simulink model "Hybrid_vehicle"  (R2020a)
settings: Solver=VariableStepAuto  StartTime=0.0  StopTime=1800  MaxStep=0.05  RelTol=1e-8
values from neighbouring files (symbols this model uses):
  Bdy_facTireFric_C = 0.018    [Model_parameters.mat]
  Bdy_lenRadiusWheel_C = 0.32    [Model_parameters.mat]
  Bdy_mEquivalentJ_C = 60    [Model_parameters.mat]
  Bdy_mVeh_C = 1400    [Model_parameters.mat]
  Bdy_vsqr2frc_C = 0.429    [Model_parameters.mat]
  Drv_facSlopeWLTC_CUR = [0 500 1000 1500 2000 2500 3000 3500 4000 4500 5000 5500 ... (98 elements, 49x2)]    [Model_parameters.mat]
  Drv_kmh2gradtqDriver_C = 200    [Model_parameters.mat]
  Drv_kmh2tqDriver_C = 500    [Model_parameters.mat]
  Drv_kmhDesWLTC_CUR = [1 2 3 4 5 6 7 8 9 10 11 12 ... (3600 elements, 1800x2)]    [Model_parameters.mat]
  Edr_pwr_LossMap_AXIS = [-150000 -100000 -60000 -35000 -23000 -7000 -2000 -1000 -200 0 200 1000 ... (19 elements, 1x19)]    [Model_parameters.mat]
  Edr_pwrInverterLosses_MAP = [19500 13000 6600 3500 2990 1470 600 450 160 50 160 450 ... (76 elements, 19x4)]    [Model_parameters.mat]
  Edr_pwrMachineLosses_MAP = [330 270 210 150 120 90 60 30 10 0 20 40 ... (209 elements, 19x11)]    [Model_parameters.mat]
  Edr_rpm_InvLossMap_AXIS = [0 2000 5000 12000]    [Model_parameters.mat]
  Edr_rpm_MachLossMap_AXIS = [0 100 200 400 1000 2000 4000 6000 8000 10000 12000]    [Model_parameters.mat]
  Edr_rpm_MaxMinTq_AXIS = [0 100 200 400 1000 2000 4000 5000 6000 7000 8000 10000 ... (13 elements, 13x1)]    [Model_parameters.mat]
  Edr_tq_MachLossMap_AXIS = [-220 -180 -140 -100 -80 -60 -40 -20 -10 0 10 20 ... (19 elements, 1x19)]    [Model_parameters.mat]
  Edr_tqEffMax_CUR = [220 220 220 220 220 220 220 180 150 125 106 81 ... (13 elements, 13x1)]    [Model_parameters.mat]
  GbxFr_tqClutchMax_C = 500    [Model_parameters.mat]
  GbxRe_facGbxReRatio_C = 10    [Model_parameters.mat]
  Ice_derfacLoadDecrease_MAP = [-5 -200 -225 -250 -275 -300 -325 -350 -375 -400 -10 -400 ... (120 elements, 10x12)]    [Model_parameters.mat]
  Ice_derfacLoadIncrease_MAP = [500 30 30 30 30 30 0 0 0 0 500 50 ... (120 elements, 10x12)]    [Model_parameters.mat]
  Ice_facEtaCocMax_MAP = [1 1 0.98 0.955 0.93 1 1 0.986 0.965 0.94 1 1 ... (35 elements, 5x7)]    [Model_parameters.mat]
  Ice_facFuelEnRich_MAP = [1 1 1 1 1 1 1 1 1 1.02 1 1 ... (35 elements, 5x7)]    [Model_parameters.mat]
  Ice_Load2TqOptIgnLamOne_MAP = [0 35 70 105 140 0 38 76 114 152 0 40 ... (35 elements, 5x7)]    [Model_parameters.mat]
  Ice_relLoad_AXIS = [0 40 80 120 160]    [Model_parameters.mat]
  Ice_relLoad_LoadDyn_AXIS = [0 80 90 100 110 120 130 140 150 160]    [Model_parameters.mat]
  Ice_relLoad_Max_CUR = [50 130 137 143 148 153 159 160 160 157 130 90]    [Model_parameters.mat]
  Ice_rpm_AXIS = [0 1000 2000 3000 4000 5000 6000]    [Model_parameters.mat]
  Ice_rpm_LoadDyn_AXIS = [500 1000 1100 1200 1300 1400 1600 2400 3000 4000 5000 6000]    [Model_parameters.mat]
  Ice_tq_AXIS = [0 40 80 120 160]    [Model_parameters.mat]
  Ice_tqLossesIce_MAP = [15 13 11 11 11 15 13 11 11 11 16 14 ... (35 elements, 5x7)]    [Model_parameters.mat]
  Ice_TqOptIgnLamOne2Load_MAP = [0 45.7 91.4 137.14 182.85 0 42.1 84.2 126.3 168.4 0 40 ... (35 elements, 5x7)]    [Model_parameters.mat]
  Pnt_capBat_C = 54000    [Model_parameters.mat]
  Pnt_facSocInit_C = 0.6    [Model_parameters.mat]
  Pnt_resBatInner_C = 0.2    [Model_parameters.mat]
libraries: simulink x2
(part 1 of 2)
settings Model: SimulationMode=accelerator  Creator=Georg  LastModifiedBy=frank
settings DataIOCC: OutputSaveName=simout  ReturnWorkspaceOutputsName=simout
settings DebuggingCC: ArithmeticOperatorsInVariantConditions=warning
settings SFSimCC: CustomCodeUndefinedFunction=UseInterfaceOnly

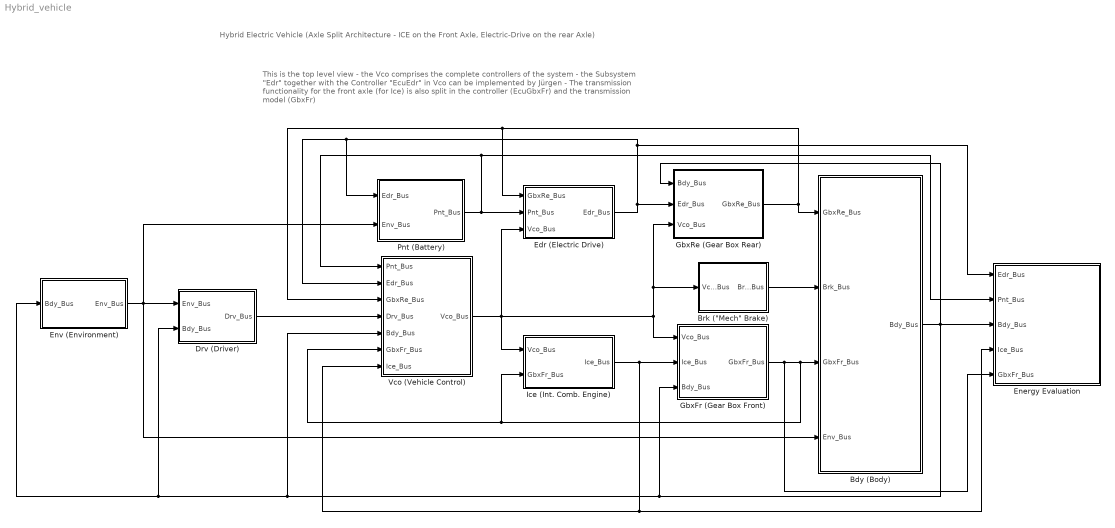
== system Hybrid_vehicle ==
  note: This is the top level view
      | - the Vco comprises the complete controllers of the system
      | - the Subsystem "Edr" together with the Controller "EcuEdr" in Vco can be implemented by Jürgen
      | - The transmission functionality for the front axle (for Ice) is also split in the controller (EcuGbxFr) and the transmission model (GbxFr)
  note: Hybrid Electric Vehicle (Axle Split Architecture - ICE on the Front Axle, Electric-Drive on the rear Axle)
  Bdy (Body) : Subsystem
      mask Display: image('Car_Top.png'); % Use "Edit Image" on toolstrip to change.
  "Brk (\"Mech\" Brake)" : Subsystem
      mask Display: image('Brakes.jpg'); % Use "Edit Image" on toolstrip to change.
  Drv (Driver) : Subsystem
      mask Display: image('Driver.jpg'); % Use "Edit Image" on toolstrip to change.
  Edr (Electric Drive) : Subsystem
      mask Display: image('e-motor.jpg'); % Use "Edit Image" on toolstrip to change.
  Energy Evaluation : Subsystem
      mask Display: image('Evaluation.png'); % Use "Edit Image" on toolstrip to change.
  Env (Environment) : Subsystem
      mask Display: image('Environment.jpg'); % Use "Edit Image" on toolstrip to change.
  GbxFr (Gear Box Front) : Subsystem
      mask Display: image('Gearbox.jpg'); % Use "Edit Image" on toolstrip to change.
  GbxRe (Gear Box Rear) : Subsystem
      mask Display: image('Gearbox.jpg'); % Use "Edit Image" on toolstrip to change.
  Ice (Int. Comb. Engine) : Subsystem
      mask Display: image('ICEngine.jpg'); % Use "Edit Image" on toolstrip to change.
  Pnt (Battery) : Subsystem
      mask Display: image('Battery.jpg'); % Use "Edit Image" on toolstrip to change.
  Vco (Vehicle Control) : Subsystem
      mask Display: image('VehicleControlUnit.jpg'); % Use "Edit Image" on toolstrip to change.
  wires:
  Drv (Driver)/1(Drv_Bus) -> Vco (Vehicle Control)/4(Drv_Bus)
  Env (Environment)/1(Env_Bus) -> Bdy (Body)/4(Env_Bus), Drv (Driver)/1(Env_Bus), Pnt (Battery)/2(Env_Bus)
  Vco (Vehicle Control)/1(Vco_Bus) -> Edr (Electric Drive)/3(Vco_Bus), Ice (Int. Comb. Engine)/1(Vco_Bus), GbxFr (Gear Box Front)/1(Vco_Bus), GbxRe (Gear Box Rear)/3(Vco_Bus), "Brk (\"Mech\" Brake)"/1(Vco_Bus)
  Pnt (Battery)/1(Pnt_Bus) -> Edr (Electric Drive)/2(Pnt_Bus), Vco (Vehicle Control)/1(Pnt_Bus), Energy Evaluation/2(Pnt_Bus)
  Edr (Electric Drive)/1(Edr_Bus) -> GbxRe (Gear Box Rear)/2(Edr_Bus), Pnt (Battery)/1(Edr_Bus), Vco (Vehicle Control)/2(Edr_Bus), Energy Evaluation/1(Edr_Bus)
  Ice (Int. Comb. Engine)/1(Ice_Bus) -> Energy Evaluation/4(Ice_Bus), Vco (Vehicle Control)/7(Ice_Bus), GbxFr (Gear Box Front)/2(Ice_Bus)
  GbxRe (Gear Box Rear)/1(GbxRe_Bus) -> Bdy (Body)/1(GbxRe_Bus), Edr (Electric Drive)/1(GbxRe_Bus), Vco (Vehicle Control)/3(GbxRe_Bus)
  GbxFr (Gear Box Front)/1(GbxFr_Bus) -> Energy Evaluation/5(GbxFr_Bus), Vco (Vehicle Control)/6(GbxFr_Bus), Ice (Int. Comb. Engine)/2(GbxFr_Bus), Bdy (Body)/3(GbxFr_Bus)
  "Brk (\"Mech\" Brake)"/1(Brk_Bus) -> Bdy (Body)/2(Brk_Bus)
  Bdy (Body)/1(Bdy_Bus) -> GbxRe (Gear Box Rear)/1(Bdy_Bus), Energy Evaluation/3(Bdy_Bus), GbxFr (Gear Box Front)/3(Bdy_Bus), Vco (Vehicle Control)/5(Bdy_Bus), Env (Environment)/1(Bdy_Bus), Drv (Driver)/2(Bdy_Bus)

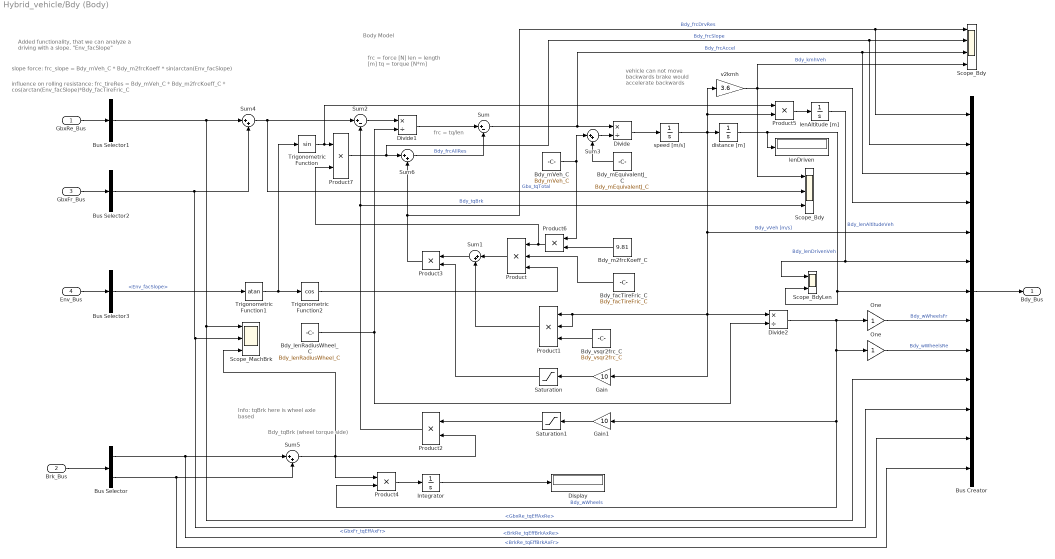
== system Hybrid_vehicle/Bdy (Body) ==
  note: influence on rolling resistance: frc_tireRes = Bdy_mVeh_C * Bdy_m2frcKoeff_C * cos(arctan(Env_facSlope)*Bdy_facTireFric_C
  note: slope force: frc_slope = Bdy_mVeh_C * Bdy_m2frcKoeff * sin(arctan(Env_facSlope)
  note: Added functionality, that we can analyze a
      | driving with a slope.  "Env_facSlope"
  note: Body Model
  note: Info:
      | tqBrk here is wheel axle based
  note: Bdy_tqBrk
      | (wheel torque side)
  note: frc = force [N]
      | len = length [m]
      | tq = torque [N*m]
  note: vehicle can not
      | move backwards
      | brake would accelerate
      | backwards
  note: frc = tq/len
  GbxRe_Bus : Inport
  Brk_Bus : Inport  Port=2
  GbxFr_Bus : Inport  Port=3
  Env_Bus : Inport  Port=4
  Bdy_facTireFric_C : Constant  Value=Bdy_facTireFric_C
  Bdy_lenRadiusWheel_C : Constant  Value=Bdy_lenRadiusWheel_C
  Bdy_m2frcKoeff_C : Constant  Value=9.81
  Bdy_mEquivalentJ_C : Constant  Value=Bdy_mEquivalentJ_C
  Bdy_mVeh_C : Constant  Value=Bdy_mVeh_C
  Bdy_vsqr2frc_C : Constant  Value=Bdy_vsqr2frc_C
  Bus Creator : BusCreator  Inputs=13
  Bus Selector : BusSelector  OutputSignals=BrkRe_tqEffBrkAxRe,BrkRe_tqEffBrkAxFr
  Bus Selector1 : BusSelector  OutputSignals=GbxRe_tqEffAxRe
  Bus Selector2 : BusSelector  OutputSignals=GbxFr_tqEffAxFr
  Bus Selector3 : BusSelector  OutputSignals=Env_facSlope
  Display : Display
  Divide : Product  Inputs=*/
  Divide1 : Product  Inputs=*/
  Divide2 : Product  Inputs=*/
  Gain : Gain  Gain=10
  Gain1 : Gain  Gain=10
  Integrator : Integrator
  One : Gain
  "One " : Gain
  Product : Product  Inputs=3  RndMeth=Zero
  Product1 : Product  Inputs=3  RndMeth=Zero
  Product2 : Product  RndMeth=Zero
  Product3 : Product  RndMeth=Zero
  Product4 : Product
  Product5 : Product
  Product6 : Product  RndMeth=Zero
  Product7 : Product
  Saturation : Saturate  UpperLimit=1  LowerLimit=-1
  Saturation1 : Saturate  UpperLimit=1  LowerLimit=-1
  Scope_Bdy : Scope  NumInputPorts=3
  "Scope_Bdy " : Scope  NumInputPorts=4
  "Scope_BdyLen  " : Scope  NumInputPorts=2
  Scope_MachBrk : Scope  NumInputPorts=3
  Sum : Sum  Inputs=|+-
  Sum{1,3..6} (5 alike) : Sum  Inputs=|++
  Sum2 : Sum  Inputs=|+-
  Trigonometric Function : Trigonometry
  Trigonometric Function1 : Trigonometry  Operator=atan
  Trigonometric Function2 : Trigonometry  Operator=cos
  distance [m] : Integrator
  lenAltitude [m] : Integrator
  lenDriven : Display
  speed [m/s] : Integrator  LimitOutput=on  LowerSaturationLimit=0
  v2kmh : Gain  Gain=3.6
  Bdy_Bus : Outport  VectorParamsAs1DForOutWhenUnconnected=off
  wires:
  Bus Creator/1 -> Bdy_Bus/1
  v2kmh/1 -> Bus Creator/4, Scope_Bdy/1, "Scope_Bdy "/4  "Bdy_kmhVeh"
  distance [m]/1 -> "Scope_BdyLen  "/2, Bus Creator/7, lenDriven/1  "Bdy_lenDrivenVeh"
  GbxFr_Bus/1 -> Bus Selector2/1
  GbxRe_Bus/1 -> Bus Selector1/1
  Brk_Bus/1 -> Bus Selector/1
  Bus Selector/1 -> Bus Creator/12, Sum5/1  "<BrkRe_tqEffBrkAxRe>"
  Bus Selector/2 -> Bus Creator/13, Sum5/2  "<BrkRe_tqEffBrkAxFr>"
  Saturation/1 -> Product3/2
  Bdy_m2frcKoeff_C/1 -> Product6/2
  Bdy_vsqr2frc_C/1 -> Product1/3
  Divide1/1 -> Sum/1
  Sum3/1 -> Divide/2
  Bdy_facTireFric_C/1 -> Product/2
  Gain/1 -> Saturation/1
  Sum/1 -> Divide/1, Bus Creator/3, "Scope_Bdy "/3  "Bdy_frcAccel"
  Gain1/1 -> Saturation1/1
  Sum5/1 -> Product2/2, Product4/1, Scope_MachBrk/3
  Sum2/1 -> Divide1/1
  Product2/1 -> Sum2/2, Scope_Bdy/3  "Bdy_tqBrk"
  Sum4/1 -> Sum2/1, Scope_Bdy/2  "Gbx_tqTotal"
  Bdy_lenRadiusWheel_C/1 -> Divide2/2, Divide1/2
  Sum1/1 -> Product3/1
  Bdy_mVeh_C/1 -> Product6/1, Sum3/1
  Product1/1 -> Sum1/2
  Divide/1 -> speed [m/s]/1
  speed [m/s]/1 -> Product5/2, v2kmh/1, distance [m]/1, Product1/1, Product1/2, Gain/1, Divide2/1, Bus Creator/5  "Bdy_vVeh [m/s]"
  Product3/1 -> Sum6/2, Bus Creator/1, "Scope_Bdy "/1  "Bdy_frcDrvRes"
  Divide2/1 -> One/1, Product4/2, Gain1/1, "One "/1  "Bdy_wWheels"
  Saturation1/1 -> Product2/1
  Bdy_mEquivalentJ_C/1 -> Sum3/2
  Bus Selector1/1 -> Sum4/1, Bus Creator/10, Scope_MachBrk/1  "<GbxRe_tqEffAxRe>"
  Bus Selector2/1 -> Sum4/2, Bus Creator/11, Scope_MachBrk/2  "<GbxFr_tqEffAxFr>"
  One/1 -> Bus Creator/9  "Bdy_wWheelsRe"
  "One "/1 -> Bus Creator/8  "Bdy_wWheelsFr"
  Product4/1 -> Integrator/1
  Integrator/1 -> Display/1
  Env_Bus/1 -> Bus Selector3/1
  Bus Selector3/1 -> Trigonometric Function1/1  "<Env_facSlope>"
  Trigonometric Function1/1 -> Trigonometric Function2/1, Trigonometric Function/1
  Trigonometric Function2/1 -> Product/3
  Sum6/1 -> Sum/2  "Bdy_frcAllRes"
  Product6/1 -> Product7/2, Product/1
  Product/1 -> Sum1/1
  Product7/1 -> Bus Creator/2, "Scope_Bdy "/2, Sum6/1  "Bdy_frcSlope"
  Trigonometric Function/1 -> Product5/1, Product7/1
  Product5/1 -> lenAltitude [m]/1
  lenAltitude [m]/1 -> "Scope_BdyLen  "/1, Bus Creator/6  "Bdy_lenAltitudeVeh"

== system Hybrid_vehicle/Brk ("Mech" Brake) ==
  note: Mechanical Brake Model
      | (both Axles)
  note: Info:
      | tq here is wheel axle based
  note: - very simple here, but a dynamik brake is not needed here
  Vco_Bus : Inport
  Bus Creator : BusCreator  Inputs=2
  Bus Selector : BusSelector  OutputSignals=EcuBrk_Bus
  Bus Selector1 : BusSelector  OutputSignals=EcuBrk_tqEffBrkAxReDes,EcuBrk_tqEffBrkAxFrDes
  Gain : Gain
  Gain1 : Gain
  Brk_Bus : Outport  VectorParamsAs1DForOutWhenUnconnected=off
  wires:
  Vco_Bus/1 -> Bus Selector/1
  Bus Selector/1 -> Bus Selector1/1  "<EcuBrk_Bus>"
  Bus Selector1/1 -> Gain/1  "<EcuBrk_tqEffBrkAxReDes>"
  Bus Selector1/2 -> Gain1/1  "<EcuBrk_tqEffBrkAxFrDes>"
  Bus Creator/1 -> Brk_Bus/1
  Gain/1 -> Bus Creator/1  "BrkRe_tqEffBrkAxRe"
  Gain1/1 -> Bus Creator/2  "BrkRe_tqEffBrkAxFr"

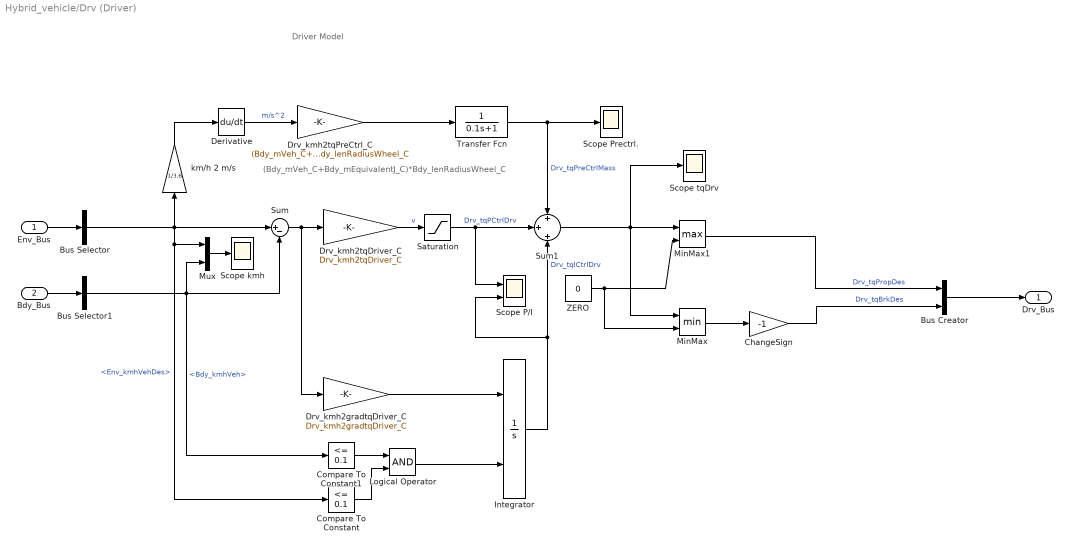
== system Hybrid_vehicle/Drv (Driver) ==
  note: (Bdy_mVeh_C+Bdy_mEquivalentJ_C)*Bdy_lenRadiusWheel_C
  note: Driver Model
  Env_Bus : Inport
  Bdy_Bus : Inport  Port=2
  Bus Creator : BusCreator  Inputs=2
  Bus Selector : BusSelector  OutputSignals=Env_kmhVehDes
  Bus Selector1 : BusSelector  OutputSignals=Bdy_kmhVeh
  ChangeSign : Gain  Gain=-1
  Compare To Constant : simulink/Logic and Bit Operations/Compare To Constant  relop=<=  const=0.1  OutDataTypeStr=boolean
  Compare To Constant1 : simulink/Logic and Bit Operations/Compare To Constant  relop=<=  const=0.1  OutDataTypeStr=boolean
  Derivative : Derivative  CoefficientInTFapproximation=0.1
  Drv_kmh2gradtqDriver_C : Gain  Gain=Drv_kmh2gradtqDriver_C
  Drv_kmh2tqDriver_C : Gain  Gain=Drv_kmh2tqDriver_C
  Drv_kmh2tqPreCtrl_C : Gain  Gain=(Bdy_mVeh_C+Bdy_mEquivalentJ_C)*Bdy_lenRadiusWheel_C
  Integrator : Integrator  ExternalReset=level  InitialCondition=-10  LimitOutput=on  UpperSaturationLimit=1000  LowerSaturationLimit=-1000
  Logical Operator : Logic  AllPortsSameDT=off  OutDataTypeStr=boolean
  MinMax : MinMax  Inputs=2
  MinMax1 : MinMax  Function=max  Inputs=2
  Mux : Mux  Inputs=2
  Saturation : Saturate  UpperLimit=1000  LowerLimit=-1000
  Scope P/I : Scope  NumInputPorts=2
  Scope Prectrl. : Scope
  Scope kmh : Scope
  Scope tqDrv : Scope
  Sum : Sum  Inputs=|+-
  Sum1 : Sum  Inputs=+|+|+
  Transfer Fcn : TransferFcn  Denominator=[0.1 1]
  ZERO : Constant  Value=0
  km/h 2 m/s : Gain  Gain=1/3.6
  Drv_Bus : Outport  VectorParamsAs1DForOutWhenUnconnected=off
  wires:
  Bus Creator/1 -> Drv_Bus/1
  MinMax1/1 -> Bus Creator/1  "Drv_tqPropDes"
  ChangeSign/1 -> Bus Creator/2  "Drv_tqBrkDes"
  Env_Bus/1 -> Bus Selector/1
  Bus Selector/1 -> Sum/1, km/h 2 m/s/1, Compare To Constant/1, Mux/1  "<Env_kmhVehDes>"
  Bdy_Bus/1 -> Bus Selector1/1
  Bus Selector1/1 -> Mux/2, Compare To Constant1/1, Sum/2  "<Bdy_kmhVeh>"
  Drv_kmh2gradtqDriver_C/1 -> Integrator/1
  ZERO/1 -> MinMax1/2, MinMax/2
  Drv_kmh2tqDriver_C/1 -> Saturation/1  "v"
  MinMax/1 -> ChangeSign/1
  Integrator/1 -> Sum1/3, Scope P/I/2  "Drv_tqICtrlDrv"
  Sum/1 -> Drv_kmh2tqDriver_C/1, Drv_kmh2gradtqDriver_C/1
  Sum1/1 -> Scope tqDrv/1, MinMax/1, MinMax1/1
  Mux/1 -> Scope kmh/1
  Derivative/1 -> Drv_kmh2tqPreCtrl_C/1  "m/s^2"
  Drv_kmh2tqPreCtrl_C/1 -> Transfer Fcn/1
  km/h 2 m/s/1 -> Derivative/1
  Transfer Fcn/1 -> Sum1/1, Scope Prectrl./1  "Drv_tqPreCtrlMass"
  Compare To Constant/1 -> Logical Operator/2
  Compare To Constant1/1 -> Logical Operator/1
  Logical Operator/1 -> Integrator/2
  Saturation/1 -> Sum1/2, Scope P/I/1  "Drv_tqPCtrlDrv"

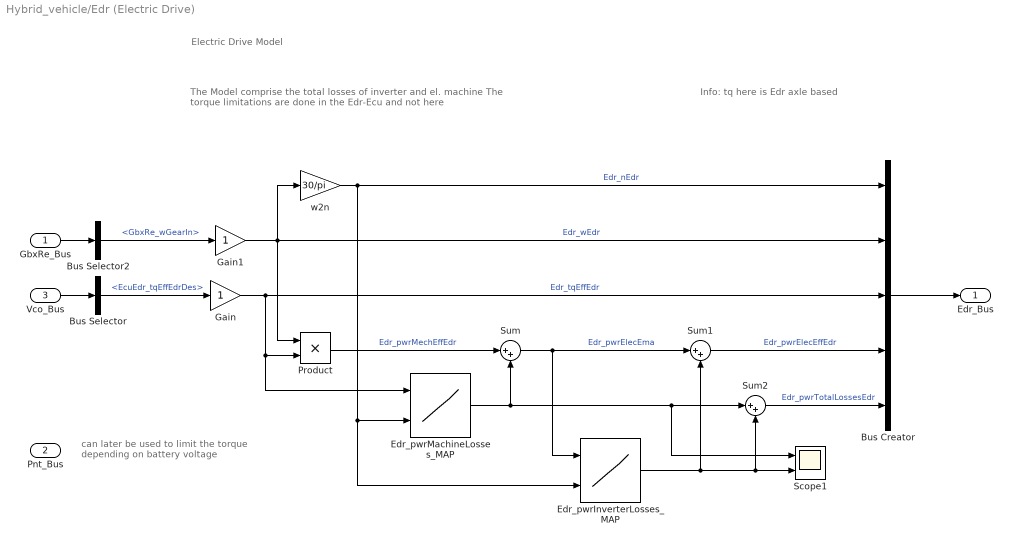
== system Hybrid_vehicle/Edr (Electric Drive) ==
  note: can later be used to limit the torque
      | depending on battery voltage
  note: Electric Drive Model
  note: Info:
      | tq here is Edr axle based
  note: The Model comprise the total losses of inverter and el. machine
      | The torque limitations are done in the Edr-Ecu and not here
  GbxRe_Bus : Inport
  Pnt_Bus : Inport  Port=2
  Vco_Bus : Inport  Port=3
  Bus Creator : BusCreator  Inputs=5
  Bus Selector : BusSelector  OutputSignals=EcuEdr_Bus.EcuEdr_tqEffEdrDes
  Bus Selector2 : BusSelector  OutputSignals=GbxRe_wGearIn
  Edr_pwrInverterLosses_MAP : Lookup_n-D  BreakpointsForDimension1=Edr_pwr_LossMap_AXIS  BreakpointsForDimension2=Edr_rpm_InvLossMap_AXIS  Table=Edr_pwrInverterLosses_MAP  ExtrapMethod=Clip  UseLastTableValue=on  InternalRulePriority=Speed  RndMeth=Simplest  InputSameDT=on
  Edr_pwrMachineLosses_MAP : Lookup_n-D  BreakpointsForDimension1=Edr_tq_MachLossMap_AXIS  BreakpointsForDimension2=Edr_rpm_MachLossMap_AXIS  Table=Edr_pwrMachineLosses_MAP  ExtrapMethod=Clip  UseLastTableValue=on  InternalRulePriority=Speed  RndMeth=Simplest  InputSameDT=on
  Gain : Gain
  Gain1 : Gain
  Product : Product
  Scope1 : Scope  NumInputPorts=2
  Sum : Sum  Inputs=|++
  Sum1 : Sum  Inputs=|++
  Sum2 : Sum  Inputs=|++
  w2n : Gain  Gain=30/pi
  Edr_Bus : Outport  VectorParamsAs1DForOutWhenUnconnected=off
  wires:
  Bus Creator/1 -> Edr_Bus/1
  Vco_Bus/1 -> Bus Selector/1
  Bus Selector/1 -> Gain/1  "<EcuEdr_tqEffEdrDes>"
  Gain/1 -> Edr_pwrMachineLosses_MAP/1, Product/2, Bus Creator/3  "Edr_tqEffEdr"
  GbxRe_Bus/1 -> Bus Selector2/1
  Bus Selector2/1 -> Gain1/1  "<GbxRe_wGearIn>"
  Gain1/1 -> Bus Creator/2, w2n/1, Product/1  "Edr_wEdr"
  w2n/1 -> Bus Creator/1, Edr_pwrInverterLosses_MAP/2, Edr_pwrMachineLosses_MAP/2  "Edr_nEdr"
  Sum1/1 -> Bus Creator/4  "Edr_pwrElecEffEdr"
  Product/1 -> Sum/1  "Edr_pwrMechEffEdr"
  Edr_pwrMachineLosses_MAP/1 -> Sum/2, Sum2/1, Scope1/1
  Sum/1 -> Sum1/1, Edr_pwrInverterLosses_MAP/1  "Edr_pwrElecEma"
  Edr_pwrInverterLosses_MAP/1 -> Sum1/2, Sum2/2, Scope1/2
  Sum2/1 -> Bus Creator/5  "Edr_pwrTotalLossesEdr"

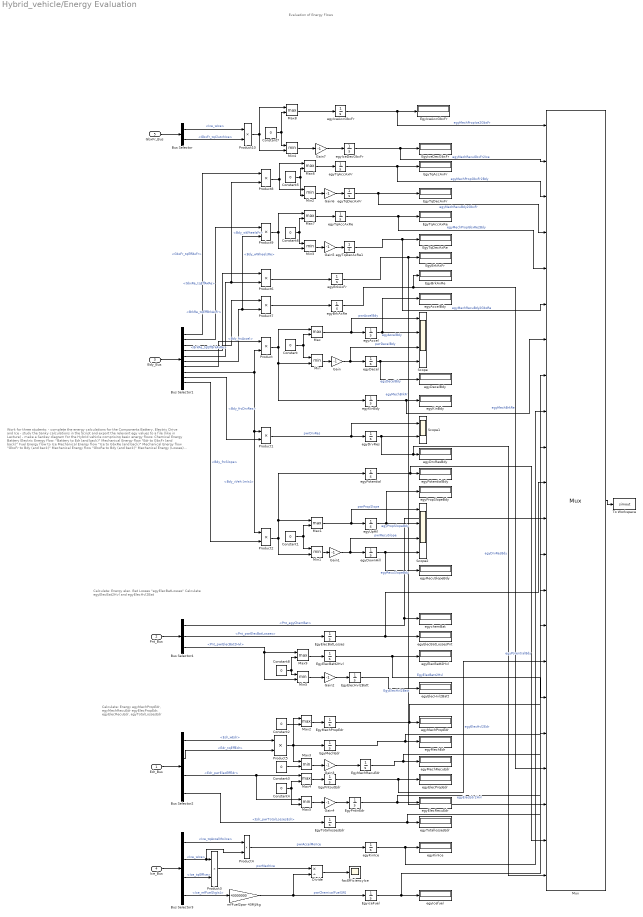
== system Hybrid_vehicle/Energy Evaluation ==
  note: Evaluation of Energy Flows
  note: Work for three students:
      | - complete the energy calculations for the Components Battery,  Electric Drive and Ice
      | - study the Sanky calculations in the Script and export the relevant egy values to a file (like in Lecture)
      | - make a Sankey diagram for the Hybrid vehicle comprising basic energy flows:
      |
      | Chemical Energy Battery
      | Electric Energy flow: "Battery to Edr (and back)"
      | Mechanical Energy flow "Edr to GbxFr (and back)"
      | Fuel Energy flow to Ice
      | Mechanical Energy flow "Ice to GbxRe (and back)"
      | Mechanical Energy flow "GbxFr to Bdy (and back)"
      | Mechanical Energy flow "GbxRe to Bdy (and back)"
      | Mechanical Energy (Losses) Brake Fr
      | Mechanical Energy (Losses) Brake Re
      | Kinetic Energy Ice
      | Kinetic Energy Bdy
      | Potential Energy Bdy
      | Show the Energies in J  (later we convert also to kWh / 100 km)
  note: Calculate: Energy elec. Bat Losses "egyElecBatLosses"
      | Calculate egyElecBat2Hvl and egyElecHvl2Bat
  note: Calculate: Energy
      | egyMechPropEdr, egyMechRecuEdr
      | egyElecPropEdr, egyElecRecuEdr,
      | egyTotalLossesEdr
  Edr_Bus : Inport
  Pnt_Bus : Inport  Port=2
  Bdy_Bus : Inport  Port=3
  Ice_Bus : Inport  Port=4
  GbxFr_Bus : Inport  Port=5
  Bus Selector : BusSelector  OutputSignals=Ice_wIce,GbxFr_tqClutchIce
  Bus Selector1 : BusSelector  OutputSignals=GbxFr_tqEffAxFr,GbxRe_tqEffAxRe,BrkRe_tqEffBrkAxRe,BrkRe_tqEffBrkAxFr,Bdy_wWheelsFr,Bdy_wWheelsRe,Bdy_frcAccel,Bdy_vVeh [m/s],Bdy_frcDrvRes,Bdy_frcSlope
  Bus Selector2 : BusSelector  OutputSignals=Edr_wEdr,Edr_tqEffEdr,Edr_pwrElecEffEdr,Edr_pwrTotalLossesEdr
  Bus Selector3 : BusSelector  OutputSignals=Ice_tqAccelMoiIce,Ice_wIce,Ice_tqEffIce,Ice_mfFuel[kg/s]
  Bus Selector4 : BusSelector  OutputSignals=Pnt_egyChemBat,Pnt_pwrElecBatLosses,Pnt_pwrElecBat2Hvl
  Constant{,1..8} (9 alike) : Constant  Value=0
  Divide : Product  Inputs=*/
  EgyBrkAxFr : Display
  EgyBrkAxRe : Display
  EgyElecBatLosses : Integrator
  EgyElecBatt2Hvl : Integrator
  EgyElecHvl2Batt : Integrator
  EgyIceAccGbxFr : Display
  EgyIceDecGbxFr : Display
  EgyMechEdr : Integrator
  EgyMechPropEdr : Integrator
  EgyMechRecuEdr : Integrator
  EgyPntinEdr : Integrator
  EgyPntoutEdr : Integrator
  EgyTotallossesEdr : Integrator
  EgyTqAccAxFr : Display
  EgyTqAccAxRe : Display
  EgyTqDecAxFr : Display
  EgyTqDecAxRe : Display
  EgyiceFuel : Integrator
  Gain{,1..7} (8 alike) : Gain  Gain=-1
  Max{,1..2,4,6..9} (8 alike) : MinMax  Function=max  Inputs=2
  Max3 : MinMax  Inputs=2
  Max5 : MinMax  Inputs=2
  Min{,1..5} (6 alike) : MinMax  Inputs=2
  Mux : Mux  Inputs=22
      settings: DisplayOption=signals
  Product{,1..10} (11 alike) : Product
  Scope : Scope  NumInputPorts=4
  Scope1 : Scope  NumInputPorts=2
  Scope2 : Scope  NumInputPorts=4
  To Workspace : ToWorkspace  VariableName=simout  SaveFormat=Structure With Time  SampleTime=-1
      settings: MaxDataPoints=1
  egyAccel : Integrator
  egyAccelBdy : Display
  egyBrkAxFr : Integrator
  egyBrkAxRe : Integrator
  egyDecel : Integrator
  egyDecelBdy : Display
  egyDownHill : Integrator
  egyDrvRes : Integrator
  "egyDrvResBdy " : Display
  egyElecBatLossesPnt : Display
  egyElecBatt2Hvl : Display
  egyElecHvl2Batt : Display
  egyElecPropEdr : Display
  egyElecRecuEdr : Display
  egyIceAccGbxFr : Integrator
  egyIceDecGbxFr : Integrator
  egyIcefuel : Display
  egyKinBdy : Integrator
  "egyKinBdy  " : Display
  egyKinIce : Integrator
  "egyKinIce " : Display
  egyMechEdr : Display
  egyMechPropEdr : Display
  egyMechRecuEdr : Display
  egyPotential : Integrator
  "egyPotentialBdy  " : Display
  egyPropSlopeBdy : Display
  egyRecuSlopeBdy : Display
  egyTotallossesEdr : Display
  egyTqAccAxFr : Integrator
  egyTqAccAxRe : Integrator
  egyTqDecAxFr : Integrator
  egyTqDecAxRe1 : Integrator
  egyUpHil : Integrator
  egychemBat : Display
  facEfficiencyIce : Scope
  mfFuel2pwr 43MJ/kg : Gain  Gain=43000000
  wires:
  Bdy_Bus/1 -> Bus Selector1/1
  Bus Selector1/8 -> Product/2, Product2/1, Product1/1  "<Bdy_vVeh [m/s]>"
  Product/1 -> egyKinBdy/1, Min/2, Max/1
  Constant/1 -> Min/1, Max/2
  Max/1 -> Scope/1, egyAccel/1  "pwrAccelBdy"
  Min/1 -> Gain/1
  Bus Selector1/7 -> Product/1  "<Bdy_frcAccel>"
  egyAccel/1 -> egyAccelBdy/1, Scope/2  "egyAccelBdy"
  egyDecel/1 -> egyDecelBdy/1, Scope/4  "egyDecelBdy"
  Gain/1 -> Scope/3, egyDecel/1  "pwrDecelBdy"
  Bus Selector1/9 -> Product1/2  "<Bdy_frcDrvRes>"
  Product1/1 -> Scope1/1, egyDrvRes/1  "pwrDrvRes"
  egyDrvRes/1 -> Mux/22, "egyDrvResBdy "/1, Scope1/2  "egyDrvResBdy"
  Bus Selector1/10 -> Product2/2  "<Bdy_frcSlope>"
  Gain1/1 -> Scope2/3, egyDownHill/1  "pwrRecuSlope"
  Constant1/1 -> Min1/1, Max1/2
  egyDownHill/1 -> egyRecuSlopeBdy/1, Scope2/4  "egyRecuSlopeBdy"
  Product2/1 -> Min1/2, egyPotential/1, Max1/1
  Min1/1 -> Gain1/1
  Max1/1 -> Scope2/1, egyUpHil/1  "pwrPropSlope"
  egyUpHil/1 -> egyPropSlopeBdy/1, Scope2/2  "egyPropSlopeBdy"
  Edr_Bus/1 -> Bus Selector2/1
  Ice_Bus/1 -> Bus Selector3/1
  Bus Selector3/4 -> mfFuel2pwr 43MJ/kg/1  "<Ice_mfFuel[kg/s]>"
  mfFuel2pwr 43MJ/kg/1 -> EgyiceFuel/1, Divide/2  "pwrChemicalFuel[W]"
  Bus Selector3/2 -> Product4/2, Product3/1  "<Ice_wIce>"
  Bus Selector3/3 -> Product3/2  "<Ice_tqEffIce>"
  Product3/1 -> Divide/1  "pwrMechIce"
  Divide/1 -> facEfficiencyIce/1
  egyKinBdy/1 -> Mux/7, "egyKinBdy  "/1
  egyPotential/1 -> Mux/21, "egyPotentialBdy  "/1  "egyPotentialBdy"
  Bus Selector3/1 -> Product4/1  "<Ice_tqAccelMoiIce>"
  Bus Selector2/1 -> Product5/1  "<Edr_wEdr>"
  Bus Selector2/2 -> Product5/2  "<Edr_tqEffEdr>"
  Bus Selector2/3 -> Max5/1, Max4/1  "<Edr_pwrElecEffEdr>"
  Product4/1 -> egyKinIce/1  "pwrAccelMoiIce"
  egyKinIce/1 -> Mux/9, "egyKinIce "/1
  Pnt_Bus/1 -> Bus Selector4/1
  Bus Selector4/2 -> EgyElecBatLosses/1  "<Pnt_pwrElecBatLosses>"
  Bus Selector4/1 -> Mux/12, egychemBat/1  "<Pnt_egyChemBat>"
  Bus Selector2/4 -> EgyTotallossesEdr/1  "<Edr_pwrTotalLossesEdr>"
  Bus Selector4/3 -> Min5/2, Max9/1  "<Pnt_pwrElecBat2Hvl>"
  EgyElecBatLosses/1 -> Mux/11, egyElecBatLossesPnt/1
  EgyElecBatt2Hvl/1 -> Mux/17, egyElecBatt2Hvl/1  "EgyElecBatt2Hvl"
  EgyElecHvl2Batt/1 -> egyElecHvl2Batt/1  "EgyElecHvl2Batt"
  Product5/1 -> Max3/1, Max2/1, EgyMechEdr/1
  EgyMechEdr/1 -> Mux/14, egyMechEdr/1
  Constant2/1 -> Max2/2
  Constant3/1 -> Max3/2
  Max2/1 -> EgyMechPropEdr/1
  Max3/1 -> Gain3/1
  EgyMechRecuEdr/1 -> Mux/15, egyMechRecuEdr/1
  EgyMechPropEdr/1 -> Mux/13, egyMechPropEdr/1
  Gain3/1 -> EgyMechRecuEdr/1
  EgyPntoutEdr/1 -> Mux/16, egyElecPropEdr/1  "egyElecHvl2Edr"
  Max4/1 -> EgyPntoutEdr/1
  Constant4/1 -> Max4/2, Max5/2
  Max5/1 -> Gain4/1
  EgyPntinEdr/1 -> Mux/18, egyElecRecuEdr/1  "egyElecEdr2Hvl"
  Gain4/1 -> EgyPntinEdr/1
  EgyTotallossesEdr/1 -> Mux/8, egyTotallossesEdr/1
  Bus Selector1/6 -> Product9/2, Product7/2  "<Bdy_wWheelsRe>"
  Bus Selector1/5 -> Product8/2, Product6/2  "<Bdy_wWheelsFr>"
  Bus Selector1/4 -> Product6/1  "<BrkRe_tqEffBrkAxFr>"
  Bus Selector1/3 -> Product7/1  "<BrkRe_tqEffBrkAxRe>"
  Product6/1 -> egyBrkAxFr/1
  Product7/1 -> egyBrkAxRe/1
  Bus Selector1/1 -> Product8/1  "<GbxFr_tqEffAxFr>"
  Bus Selector1/2 -> Product9/1  "<GbxRe_tqEffAxRe>"
  Product8/1 -> Min2/1, Max6/1
  egyTqAccAxRe/1 -> Mux/5, EgyTqAccAxRe/1  "egyMechPropGbxRe2Bdy"
  Constant5/1 -> Max6/2, Min2/2
  Max6/1 -> egyTqAccAxFr/1
  Min2/1 -> Gain6/1
  egyTqDecAxFr/1 -> Mux/4, EgyTqDecAxFr/1  "egyMechRecuBdy2GbxFr"
  Constant6/1 -> Max7/2, Min3/1
  Product9/1 -> Max7/1, Min3/2
  Max7/1 -> egyTqAccAxRe/1
  Min3/1 -> Gain5/1
  egyTqDecAxRe1/1 -> Mux/6, EgyTqDecAxRe/1  "egyMechRecuBdy2GbxRe"
  GbxFr_Bus/1 -> Bus Selector/1
  Bus Selector/2 -> Product10/2  "<GbxFr_tqClutchIce>"
  Bus Selector/1 -> Product10/1  "<Ice_wIce>"
  Constant7/1 -> Min4/1, Max8/2
  Product10/1 -> Min4/2, Max8/1
  Gain5/1 -> egyTqDecAxRe1/1
  Gain6/1 -> egyTqDecAxFr/1
  Max8/1 -> egyIceAccGbxFr/1
  Min4/1 -> Gain7/1
  Gain7/1 -> egyIceDecGbxFr/1
  egyIceDecGbxFr/1 -> Mux/2, EgyIceDecGbxFr/1  "egyMechRecuGbxFr2Ice"
  egyIceAccGbxFr/1 -> Mux/1, EgyIceAccGbxFr/1  "egyMechPropIce2GbxFr"
  EgyiceFuel/1 -> Mux/10, egyIcefuel/1
  egyTqAccAxFr/1 -> Mux/3, EgyTqAccAxFr/1  "egyMechPropGbxFr2Bdy"
  egyBrkAxRe/1 -> Mux/19, EgyBrkAxRe/1  "egyMechBrkRe"
  egyBrkAxFr/1 -> Mux/20, EgyBrkAxFr/1  "egyMechBrkFr"
  Mux/1 -> To Workspace/1
  Constant8/1 -> Max9/2, Min5/1
  Min5/1 -> Gain2/1
  Gain2/1 -> EgyElecHvl2Batt/1
  Max9/1 -> EgyElecBatt2Hvl/1

== system Hybrid_vehicle/Env (Environment) ==
  note: Environment Model
  Bdy_Bus : Inport
  Bus Creator : BusCreator  Inputs=2
  Bus Selector1 : BusSelector  OutputSignals=Bdy_lenDrivenVeh
  Clock : Clock
  Derivative1 : Derivative  CoefficientInTFapproximation=0.1
  Drv_facSlopeWLTC_24000m_CUR : Lookup  InputValues=Drv_facSlopeWLTC_CUR(:,1)  Table=Drv_facSlopeWLTC_CUR(:,2)  LookUpMeth=Interpolation-Use End Values
  Drv_kmhDesWLTC_1800s_CUR : Lookup  InputValues=Drv_kmhDesWLTC_CUR(:,1)  Table=Drv_kmhDesWLTC_CUR(:,2)  LookUpMeth=Interpolation-Use End Values
  Integrator2 : Integrator  UpperSaturationLimit=200.0001  LowerSaturationLimit=199.9999
  Mux : Mux  Inputs=2
  Scope kmhDesFil : Scope
  Slope as a factor 0.1 means 10 m climb on a basis of 100 m Angle alfa = arctan(facSlope) : Constant  Value=0.1
  Transfer Fcn1 : TransferFcn  Denominator=[0.4 1]
  Transfer Fcn2 : TransferFcn  Denominator=[0.4 1]
  Env_Bus : Outport  VectorParamsAs1DForOutWhenUnconnected=off
  wires:
  Bus Creator/1 -> Env_Bus/1
  Drv_kmhDesWLTC_1800s_CUR/1 -> Mux/1, Derivative1/1
  Drv_facSlopeWLTC_24000m_CUR/1 -> Bus Creator/2  "Env_facSlope"
  Clock/1 -> Drv_kmhDesWLTC_1800s_CUR/1
  Integrator2/1 -> Mux/2, Bus Creator/1  "Env_kmhVehDes"
  Mux/1 -> Scope kmhDesFil/1
  Derivative1/1 -> Transfer Fcn1/1
  Transfer Fcn1/1 -> Transfer Fcn2/1
  Transfer Fcn2/1 -> Integrator2/1
  Bdy_Bus/1 -> Bus Selector1/1
  Bus Selector1/1 -> Drv_facSlopeWLTC_24000m_CUR/1  "<Bdy_lenDrivenVeh>"

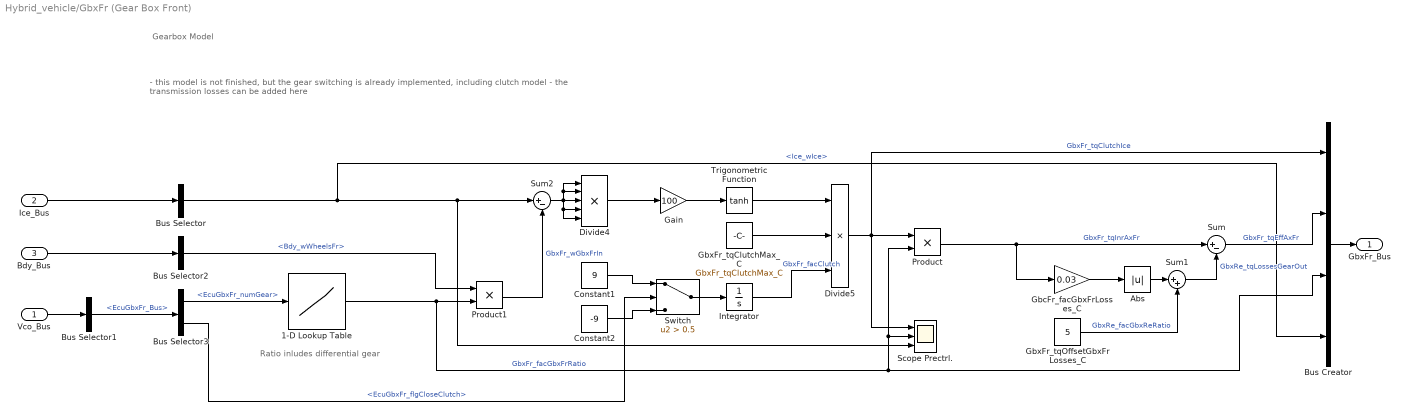
== system Hybrid_vehicle/GbxFr (Gear Box Front) ==
  note: Ratio inludes differential gear
  note: Gearbox Model
  note: - this model is not finished, but the gear switching is already implemented, including clutch model
      | - the transmission losses can be added here
  Vco_Bus : Inport
  Ice_Bus : Inport  Port=2
  Bdy_Bus : Inport  Port=3
  1-D Lookup Table : Lookup_n-D  NumberOfTableDimensions=1  BreakpointsForDimension1=[1 2 3 4 5]  Table="[12.144\t7.155392\t4.812336\t3.788192\t3.080896]"  InterpMethod=Nearest  InternalRulePriority=Speed  RndMeth=Simplest  InputSameDT=on
  Abs : Abs
  Bus Creator : BusCreator  Inputs=4
  Bus Selector : BusSelector  OutputSignals=Ice_wIce
  Bus Selector1 : BusSelector  OutputSignals=EcuGbxFr_Bus
  Bus Selector2 : BusSelector  OutputSignals=Bdy_wWheelsFr
  Bus Selector3 : BusSelector  OutputSignals=EcuGbxFr_numGear,EcuGbxFr_flgCloseClutch
  Constant1 : Constant  Value=9
  Constant2 : Constant  Value=-9
  Divide4 : Product  Inputs=*****
  Divide5 : Product  Inputs=***
  Gain : Gain  Gain=100
  GbcFr_facGbxFrLosses_C : Gain  Gain=0.03
  GbxFr_tqClutchMax_C : Constant  Value=GbxFr_tqClutchMax_C
  GbxFr_tqOffsetGbxFrLosses_C : Constant  Value=5
  Integrator : Integrator  LimitOutput=on  UpperSaturationLimit=1  LowerSaturationLimit=0
  Product : Product
  Product1 : Product
  Scope Prectrl. : Scope  NumInputPorts=3
  Sum : Sum  Inputs=|+-
  Sum1 : Sum  Inputs=|++
  Sum2 : Sum  Inputs=|+-
  Switch : Switch  Criteria=u2 > Threshold  Threshold=0.5
  Trigonometric Function : Trigonometry  Operator=tanh
  GbxFr_Bus : Outport  VectorParamsAs1DForOutWhenUnconnected=off
  wires:
  Vco_Bus/1 -> Bus Selector1/1
  Ice_Bus/1 -> Bus Selector/1
  Bdy_Bus/1 -> Bus Selector2/1
  Bus Creator/1 -> GbxFr_Bus/1
  1-D Lookup Table/1 -> Product1/2, Product/2, Scope Prectrl./2, Bus Creator/3  "GbxFr_facGbxFrRatio"
  Sum/1 -> Bus Creator/2  "GbxFr_tqEffAxFr"
  Bus Selector/1 -> Bus Creator/4, Sum2/1, Scope Prectrl./3  "<Ice_wIce>"
  Bus Selector2/1 -> Product1/1  "<Bdy_wWheelsFr>"
  Divide5/1 -> Product/1, Bus Creator/1, Scope Prectrl./1  "GbxFr_tqClutchIce"
  Bus Selector1/1 -> Bus Selector3/1  "<EcuGbxFr_Bus>"
  Bus Selector3/1 -> 1-D Lookup Table/1  "<EcuGbxFr_numGear>"
  Product1/1 -> Sum2/2  "GbxFr_wGbxFrIn"
  Sum2/1 -> Divide4/5, Divide4/4, Divide4/1, Divide4/2, Divide4/3
  Divide4/1 -> Gain/1
  Gain/1 -> Trigonometric Function/1
  GbxFr_tqClutchMax_C/1 -> Divide5/2
  Trigonometric Function/1 -> Divide5/1
  Constant1/1 -> Switch/1
  Constant2/1 -> Switch/3
  Switch/1 -> Integrator/1
  Integrator/1 -> Divide5/3  "GbxFr_facClutch"
  Bus Selector3/2 -> Switch/2  "<EcuGbxFr_flgCloseClutch>"
  Abs/1 -> Sum1/1
  GbxFr_tqOffsetGbxFrLosses_C/1 -> Sum1/2  "GbxRe_facGbxReRatio"
  Sum1/1 -> Sum/2  "GbxRe_tqLossesGearOut"
  GbcFr_facGbxFrLosses_C/1 -> Abs/1
  Product/1 -> GbcFr_facGbxFrLosses_C/1, Sum/1  "GbxFr_tqInrAxFr"

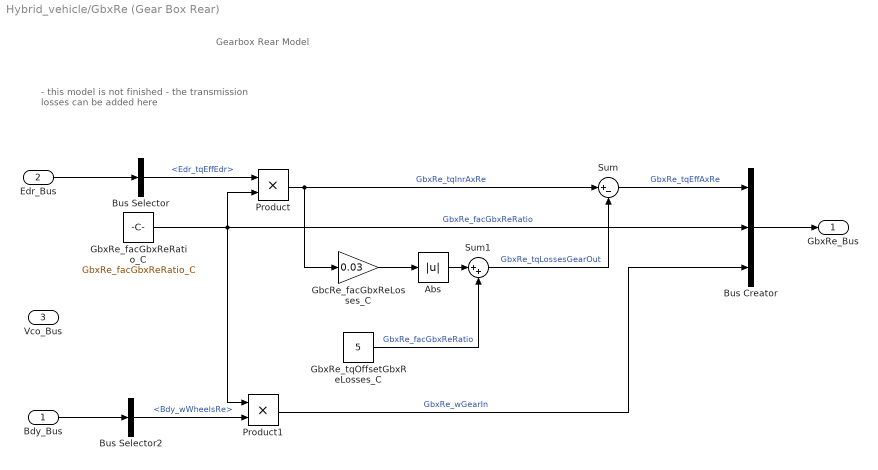
== system Hybrid_vehicle/GbxRe (Gear Box Rear) ==
  note: Gearbox Rear Model
  note: - this model is not finished
      | - the transmission losses can be added here
  Bdy_Bus : Inport
  Edr_Bus : Inport  Port=2
  Vco_Bus : Inport  Port=3
  Abs : Abs
  Bus Creator : BusCreator  Inputs=3
  Bus Selector : BusSelector  OutputSignals=Edr_tqEffEdr
  Bus Selector2 : BusSelector  OutputSignals=Bdy_wWheelsRe
  GbcRe_facGbxReLosses_C : Gain  Gain=0.03
  GbxRe_facGbxReRatio_C : Constant  Value=GbxRe_facGbxReRatio_C
  GbxRe_tqOffsetGbxReLosses_C : Constant  Value=5
  Product : Product
  Product1 : Product
  Sum : Sum  Inputs=|+-
  Sum1 : Sum  Inputs=|++
  GbxRe_Bus : Outport  VectorParamsAs1DForOutWhenUnconnected=off
  wires:
  Edr_Bus/1 -> Bus Selector/1
  Bdy_Bus/1 -> Bus Selector2/1
  Bus Creator/1 -> GbxRe_Bus/1
  Bus Selector/1 -> Product/1  "<Edr_tqEffEdr>"
  Product/1 -> Sum/1, GbcRe_facGbxReLosses_C/1  "GbxRe_tqInrAxRe"
  GbxRe_facGbxReRatio_C/1 -> Bus Creator/2, Product/2, Product1/1  "GbxRe_facGbxReRatio"
  Bus Selector2/1 -> Product1/2  "<Bdy_wWheelsRe>"
  Product1/1 -> Bus Creator/3  "GbxRe_wGearIn"
  Sum/1 -> Bus Creator/1  "GbxRe_tqEffAxRe"
  Sum1/1 -> Sum/2  "GbxRe_tqLossesGearOut"
  GbxRe_tqOffsetGbxReLosses_C/1 -> Sum1/2  "GbxRe_facGbxReRatio"
  GbcRe_facGbxReLosses_C/1 -> Abs/1
  Abs/1 -> Sum1/1

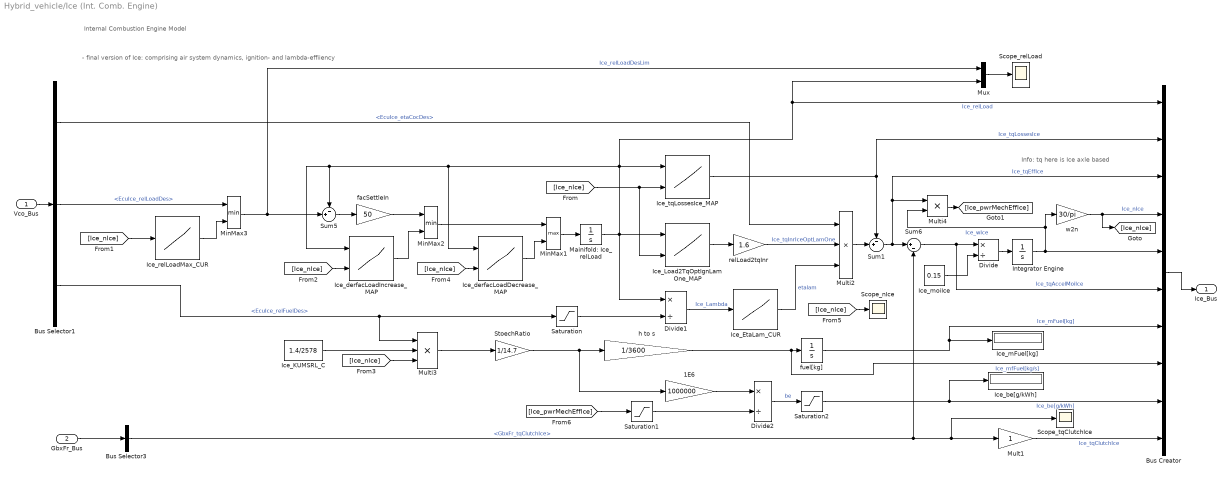
== system Hybrid_vehicle/Ice (Int. Comb. Engine) ==
  note: Internal Combustion Engine Model
  note: Info:
      | tq here is Ice axle based
  note: - final version of Ice: comprising air system dynamics, ignition- and lambda-effiiency
  Vco_Bus : Inport
  GbxFr_Bus : Inport  Port=2
  " h to s" : Gain  Gain=1/3600
  1E6 : Gain  Gain=1000000
  Bus Creator : BusCreator  Inputs=10
  Bus Selector1 : BusSelector  OutputSignals=EcuIce_Bus.EcuIce_etaCocDes,EcuIce_Bus.EcuIce_relLoadDes,EcuIce_Bus.EcuIce_relFuelDes
  Bus Selector3 : BusSelector  OutputSignals=GbxFr_tqClutchIce
  Divide : Product  Inputs=*/
  Divide1 : Product  Inputs=*/
  Divide2 : Product  Inputs=*/
  Ice_EtaLam_CUR : Lookup_n-D  NumberOfTableDimensions=1  BreakpointsForDimension1="[0.5    0.6     0.7   0.8   0.85   0.9   1.0   1.1    1.2    1.3    1.4    1.5    1.6    1.7    1.8    1.9    2.0]"  Table="[0       0.5       1     1.1  1.12  1.06   1.0  0.93  0.85   0.78   0.72    0.66    0.625   0.588  0.3  0.2  0]"  ExtrapMethod=Clip  InternalRulePriority=Speed  RndMeth=Simplest  InputSameDT=on
  Ice_KUMSRL_C : Constant  Value=1.4/2578
  Ice_Load2TqOptIgnLamOne_MAP : Lookup_n-D  BreakpointsForDimension1=Ice_relLoad_AXIS  BreakpointsForDimension2=Ice_rpm_AXIS  Table=Ice_Load2TqOptIgnLamOne_MAP  ExtrapMethod=Clip  InternalRulePriority=Speed  RndMeth=Simplest  InputSameDT=on
  Ice_be[g/kWh] : Display
  Ice_derfacLoadDecrease_MAP : Lookup_n-D  BreakpointsForDimension1=Ice_relLoad_LoadDyn_AXIS  BreakpointsForDimension2=Ice_rpm_LoadDyn_AXIS  Table=Ice_derfacLoadDecrease_MAP  ExtrapMethod=Clip  UseLastTableValue=on  InternalRulePriority=Speed  RndMeth=Simplest  InputSameDT=on
  Ice_derfacLoadIncrease_MAP : Lookup_n-D  BreakpointsForDimension1=Ice_relLoad_LoadDyn_AXIS  BreakpointsForDimension2=Ice_rpm_LoadDyn_AXIS  Table=Ice_derfacLoadIncrease_MAP  ExtrapMethod=Clip  UseLastTableValue=on  InternalRulePriority=Speed  RndMeth=Simplest  InputSameDT=on
  Ice_mFuel[kg] : Display
  Ice_moiIce : Constant  Value=0.15
  Ice_relLoadMax_CUR : Lookup_n-D  NumberOfTableDimensions=1  BreakpointsForDimension1=Ice_rpm_LoadDyn_AXIS  Table=Ice_relLoad_Max_CUR  ExtrapMethod=Clip  InternalRulePriority=Speed  RndMeth=Simplest  InputSameDT=on
  Ice_tqLossesIce_MAP : Lookup_n-D  BreakpointsForDimension1=Ice_relLoad_AXIS  BreakpointsForDimension2=Ice_rpm_AXIS  Table=Ice_tqLossesIce_MAP  ExtrapMethod=Clip  InternalRulePriority=Speed  RndMeth=Simplest  InputSameDT=on
  Integrator Engine : Integrator  LimitOutput=on  LowerSaturationLimit=0
  Mainifold: Ice_relLoad : Integrator  InitialCondition=80  LimitOutput=on  LowerSaturationLimit=0
  MinMax1 : MinMax  Function=max  Inputs=2
  MinMax2 : MinMax  Inputs=2
  MinMax3 : MinMax  Inputs=2
  Mult1 : Gain
  Multi2 : Product  Inputs=***
  Multi3 : Product  Inputs=***
  Multi4 : Product  Inputs=**
  Mux : Mux  Inputs=2
  Saturation : Saturate  UpperLimit=1000  LowerLimit=0.0001
  Saturation1 : Saturate  UpperLimit=10000000  LowerLimit=0.1
  Saturation2 : Saturate  UpperLimit=1000  LowerLimit=0
  Scope_nIce : Scope
  Scope_relLoad : Scope
  Scope_tqClutchIce : Scope
  StoechRatio : Gain  Gain=1/14.7
  Sum1 : Sum  Inputs=-+|
  Sum5 : Sum  Inputs=-+|
  Sum6 : Sum  Inputs=|+-
  facSettleIn : Gain  Gain=50
  fuel[kg] : Integrator
  relLoad2tqInr : Gain  Gain=1.6
  w2n : Gain  Gain=30/pi
  Ice_Bus : Outport  VectorParamsAs1DForOutWhenUnconnected=off
  wires:
  Bus Creator/1 -> Ice_Bus/1
  Bus Selector1/2 -> MinMax3/1  "<EcuIce_relLoadDes>"
  Vco_Bus/1 -> Bus Selector1/1
  Divide/1 -> Integrator Engine/1
  Ice_moiIce/1 -> Divide/2
  Bus Selector3/1 -> Scope_tqClutchIce/1, Mult1/1, Sum6/2  "<GbxFr_tqClutchIce>"
  Integrator Engine/1 -> Bus Creator/5, w2n/1, Multi4/2  "Ice_wIce"
  GbxFr_Bus/1 -> Bus Selector3/1
  Mainifold: Ice_relLoad/1 -> Divide1/1, Mux/2, Bus Creator/1, Ice_derfacLoadIncrease_MAP/1, Sum5/1, Ice_derfacLoadDecrease_MAP/1, Ice_tqLossesIce_MAP/1, Ice_Load2TqOptIgnLamOne_MAP/1  "Ice_relLoad"
  w2n/1 -> Bus Creator/4, [Ice_nIce]  "Ice_nIce"
  Ice_tqLossesIce_MAP/1 -> Sum1/1, Bus Creator/2  "Ice_tqLossesIce"
  relLoad2tqInr/1 -> Multi2/2  "Ice_tqInrIceOptLamOne"
  Sum1/1 -> Bus Creator/3, Multi4/1, Sum6/1  "Ice_tqEffIce"
  Ice_relLoadMax_CUR/1 -> MinMax3/2
  MinMax1/1 -> Mainifold: Ice_relLoad/1
  Ice_derfacLoadDecrease_MAP/1 -> MinMax1/2
  MinMax2/1 -> MinMax1/1
  Ice_derfacLoadIncrease_MAP/1 -> MinMax2/2
  facSettleIn/1 -> MinMax2/1
  Sum5/1 -> facSettleIn/1
  MinMax3/1 -> Sum5/2, Mux/1  "Ice_relLoadDesLim"
  Mux/1 -> Scope_relLoad/1
  Ice_Load2TqOptIgnLamOne_MAP/1 -> relLoad2tqInr/1
  [Ice_nIce] -> Ice_Load2TqOptIgnLamOne_MAP/2, Ice_tqLossesIce_MAP/2
  [Ice_nIce] -> Ice_relLoadMax_CUR/1
  [Ice_nIce] -> Ice_derfacLoadIncrease_MAP/2
  [Ice_nIce] -> Ice_derfacLoadDecrease_MAP/2
  Multi2/1 -> Sum1/2
  Bus Selector1/3 -> Multi3/1, Saturation/1  "<EcuIce_relFuelDes>"
  Divide1/1 -> Ice_EtaLam_CUR/1  "Ice_Lambda"
  Saturation/1 -> Divide1/2
  Ice_EtaLam_CUR/1 -> Multi2/3  "etalam"
  Bus Selector1/1 -> Multi2/1  "<EcuIce_etaCocDes>"
  Multi3/1 -> StoechRatio/1
  Ice_KUMSRL_C/1 -> Multi3/2
  [Ice_nIce] -> Multi3/3
  StoechRatio/1 -> 1E6/1, " h to s"/1
  " h to s"/1 -> Bus Creator/8, fuel[kg]/1  "Ice_mfFuel[kg/s]"
  [Ice_nIce] -> Scope_nIce/1
  fuel[kg]/1 -> Bus Creator/7, Ice_mFuel[kg]/1  "Ice_mFuel[kg]"
  Multi4/1 -> [Ice_pwrMechEffIce]
  1E6/1 -> Divide2/1
  [Ice_pwrMechEffIce] -> Saturation1/1
  Saturation1/1 -> Divide2/2
  Divide2/1 -> Saturation2/1  "be"
  Saturation2/1 -> Ice_be[g/kWh]/1, Bus Creator/9  "Ice_be[g/kWh]"
  Sum6/1 -> Bus Creator/6, Divide/1  "Ice_tqAccelMoiIce"
  Mult1/1 -> Bus Creator/10  "Ice_tqClutchIce"

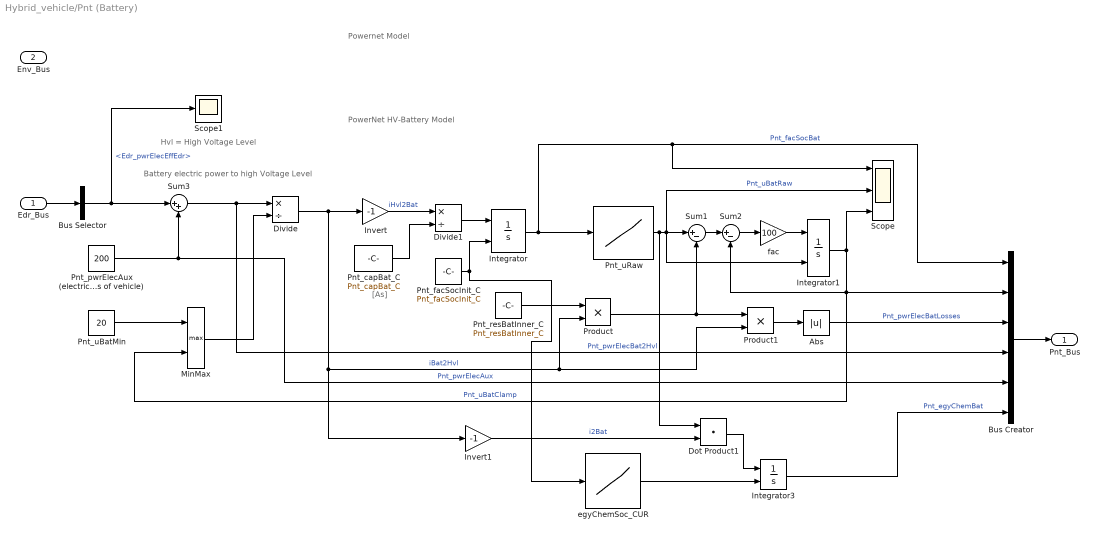
== system Hybrid_vehicle/Pnt (Battery) ==
  note: Hvl = High Voltage Level
  note: Battery electric power to high Voltage Level
  note: Powernet Model
  note: PowerNet HV-Battery Model
  note: [As]
  Edr_Bus : Inport
  Env_Bus : Inport  Port=2
  Abs : Abs
  Bus Creator : BusCreator  Inputs=6
  Bus Selector : BusSelector  OutputSignals=Edr_pwrElecEffEdr
  Divide : Product  Inputs=*/
  Divide1 : Product  Inputs=*/
  Dot Product1 : DotProduct  InputSameDT=on  OutDataTypeStr=Inherit: Inherit via internal rule
  Integrator : Integrator  InitialConditionSource=external  InitialCondition=0.8  LimitOutput=on  UpperSaturationLimit=1  LowerSaturationLimit=0
  Integrator1 : Integrator  InitialConditionSource=external  InitialCondition=0.8
  Integrator3 : Integrator  InitialConditionSource=external
  Invert : Gain  Gain=-1
  Invert1 : Gain  Gain=-1
  MinMax : MinMax  Function=max  Inputs=2
  Pnt_capBat_C : Constant  Value=Pnt_capBat_C
  Pnt_facSocInit_C : Constant  Value=Pnt_facSocInit_C
  Pnt_pwrElecAux (electric auxilliaries of vehicle) : Constant  Value=200
  Pnt_resBatInner_C : Constant  Value=Pnt_resBatInner_C
  Pnt_uBatMin : Constant  Value=20
  Pnt_uRaw : Lookup  InputValues="[0, 0.1 0.2  0.5  0.8  1]"  Table="[50 250  290   350  385  400]"  LookUpMeth=Interpolation-Use End Values
  Product : Product  RndMeth=Zero
  Product1 : Product  RndMeth=Zero
  Scope : Scope  NumInputPorts=3
  Scope1 : Scope
  Sum1 : Sum  Inputs=|+-
  Sum2 : Sum  Inputs=|+-
  Sum3 : Sum  Inputs=|++
  egyChemSoc_CUR : Lookup_n-D  NumberOfTableDimensions=1  BreakpointsForDimension1=[0 0.05 0.1 0.2 0.3 0.4 0.5 0.6 0.7 0.8 0.9 1]  Table=[0 2.751 8.13 22.73 38.87 56.19 74.6 93.75 113.6 134.2 155.1 176.5 ]*10^5  InternalRulePriority=Speed  RndMeth=Simplest  InputSameDT=on
  fac : Gain  Gain=100
  Pnt_Bus : Outport  VectorParamsAs1DForOutWhenUnconnected=off
  wires:
  Bus Creator/1 -> Pnt_Bus/1
  Edr_Bus/1 -> Bus Selector/1
  Integrator1/1 -> Scope/3, Sum2/2, Bus Creator/2, MinMax/2  "Pnt_uBatClamp"
  Invert/1 -> Divide1/1  "iHvl2Bat"
  Pnt_resBatInner_C/1 -> Product/1
  MinMax/1 -> Divide/2
  Bus Selector/1 -> Sum3/1, Scope1/1  "<Edr_pwrElecEffEdr>"
  Product/1 -> Sum1/2, Product1/1
  Sum1/1 -> Sum2/1
  Pnt_capBat_C/1 -> Divide1/2
  Divide1/1 -> Integrator/1
  Integrator/1 -> Pnt_uRaw/1, Bus Creator/1, Scope/1  "Pnt_facSocBat"
  Pnt_uBatMin/1 -> MinMax/1
  Product1/1 -> Abs/1
  Abs/1 -> Bus Creator/3  "Pnt_pwrElecBatLosses"
  Sum2/1 -> fac/1
  fac/1 -> Integrator1/1
  Sum3/1 -> Bus Creator/4, Divide/1  "Pnt_pwrElecBat2Hvl"
  Pnt_pwrElecAux (electric auxilliaries of vehicle)/1 -> Bus Creator/5, Sum3/2  "Pnt_pwrElecAux"
  Invert1/1 -> Dot Product1/2  "i2Bat"
  Pnt_uRaw/1 -> Dot Product1/1, Scope/2, Integrator1/2, Sum1/1  "Pnt_uBatRaw"
  Pnt_facSocInit_C/1 -> Integrator/2, egyChemSoc_CUR/1
  egyChemSoc_CUR/1 -> Integrator3/2
  Dot Product1/1 -> Integrator3/1
  Divide/1 -> Invert/1, Invert1/1, Product/2, Product1/2  "iBat2Hvl"
  Integrator3/1 -> Bus Creator/6  "Pnt_egyChemBat"

== system Hybrid_vehicle/Vco (Vehicle Control) ==
  note: Vehicle Control Model
  Pnt_Bus : Inport
  Edr_Bus : Inport  Port=2
  GbxRe_Bus : Inport  Port=3
  Drv_Bus : Inport  Port=4
  Bdy_Bus : Inport  Port=5
  GbxFr_Bus : Inport  Port=6
  Ice_Bus : Inport  Port=7
  Bus Creator : BusCreator  Inputs=5
  EcuBrk (Electronic Control Unit for Brakes) : Subsystem
  EcuEdr (Electronic Control Unit for Edr) : Subsystem
  EcuGbxFr (Electronic Control Unit for Gbx Front) : Subsystem
  EcuGbxRe (Electronic Control Unit for Gbx Rear) : Subsystem
  EcuIce (Electronic Control Unit for Ice) : Subsystem
  Vec (Vehicle Coordination) : Subsystem
  Vco_Bus : Outport  VectorParamsAs1DForOutWhenUnconnected=off
  wires:
  Bus Creator/1 -> Vco_Bus/1
  EcuIce (Electronic Control Unit for Ice)/1(EcuIce_Bus) -> Bus Creator/3  "EcuIce_Bus"
  EcuGbxFr (Electronic Control Unit for Gbx Front)/2(EcuGbxFr_Bus) -> Bus Creator/4  "EcuGbxFr_Bus"
  EcuEdr (Electronic Control Unit for Edr)/1(EcuEdr_Bus) -> Bus Creator/1  "EcuEdr_Bus"
  EcuGbxFr (Electronic Control Unit for Gbx Front)/1(EcuGbxFr_tqEffIceDes) -> EcuIce (Electronic Control Unit for Ice)/4(EcuGbxFr_tqEffIceDes)
  EcuGbxRe (Electronic Control Unit for Gbx Rear)/1(EcuGbxRe_tqEffEdrDes) -> EcuEdr (Electronic Control Unit for Edr)/2(EcuGbxRe_tqEffEdrDes)
  EcuGbxRe (Electronic Control Unit for Gbx Rear)/2(EcuGbxRe_Bus) -> Bus Creator/2  "EcuGbxRe_Bus"
  Drv_Bus/1 -> Vec (Vehicle Coordination)/3(Drv_Bus)
  Pnt_Bus/1 -> Vec (Vehicle Coordination)/4(Pnt_Bus)
  Edr_Bus/1 -> Vec (Vehicle Coordination)/1(Edr_Bus)
  GbxFr_Bus/1 -> Vec (Vehicle Coordination)/5(GbxFr_Bus)
  Ice_Bus/1 -> Vec (Vehicle Coordination)/2(Ice_Bus)
  EcuBrk (Electronic Control Unit for Brakes)/1(EcuBrk_Bus) -> Bus Creator/5  "EcuBrk_Bus"
  Vec (Vehicle Coordination)/2(Vec_tqEffAxReDes) -> EcuGbxRe (Electronic Control Unit for Gbx Rear)/1(Vec_tqEffAxReDes)
  Vec (Vehicle Coordination)/7(Vec_tqEffAxFrDes) -> EcuGbxFr (Electronic Control Unit for Gbx Front)/2(Vec_tqEffAxFrDes)
  GbxRe_Bus/1 -> Vec (Vehicle Coordination)/6(GbxRe_Bus)
  Vec (Vehicle Coordination)/8(GbxFr_facGbxFrRatio) -> EcuGbxFr (Electronic Control Unit for Gbx Front)/3(GbxFr_facGbxFrRatio)
  Vec (Vehicle Coordination)/3(GbxRe_facGbxReRatio) -> EcuGbxRe (Electronic Control Unit for Gbx Rear)/2(GbxRe_facGbxReRatio)
  Vec (Vehicle Coordination)/10(Vec_tqEffBrkAxReDes) -> EcuBrk (Electronic Control Unit for Brakes)/1(Vec_tqEffBrkAxReDes)
  Vec (Vehicle Coordination)/11(Vec_tqEffBrkAxFrDes) -> EcuBrk (Electronic Control Unit for Brakes)/2(Vec_tqEffBrkAxFrDes)
  Bdy_Bus/1 -> Vec (Vehicle Coordination)/7(Bdy_Bus)
  Vec (Vehicle Coordination)/9(Bdy_kmhVeh) -> EcuGbxFr (Electronic Control Unit for Gbx Front)/4(Bdy_kmhVeh)
  Vec (Vehicle Coordination)/1(Edr_nEdr) -> EcuEdr (Electronic Control Unit for Edr)/1(Edr_nEdr)
  Vec (Vehicle Coordination)/4(Ice_relLoad) -> EcuIce (Electronic Control Unit for Ice)/1(Ice_relLoad)
  Vec (Vehicle Coordination)/5(Ice_nIce) -> EcuIce (Electronic Control Unit for Ice)/2(Ice_nIce)
  Vec (Vehicle Coordination)/6(Vec_flgIceOn) -> EcuIce (Electronic Control Unit for Ice)/3(Vec_flgIceOn), EcuGbxFr (Electronic Control Unit for Gbx Front)/1(Vec_flgIceOn)

== system Hybrid_vehicle/Vco (Vehicle Control)/EcuBrk (Electronic Control Unit for Brakes) ==
  note: Info:
      | tq here is wheel axle based
  note: Vehicle Control Unit for Brakes
  Vec_tqEffBrkAxReDes : Inport
  Vec_tqEffBrkAxFrDes : Inport  Port=2
  Bus Creator : BusCreator  Inputs=2
  EcuBrk_Bus : Outport  VectorParamsAs1DForOutWhenUnconnected=off
  wires:
  Vec_tqEffBrkAxReDes/1 -> Bus Creator/1  "EcuBrk_tqEffBrkAxReDes"
  Vec_tqEffBrkAxFrDes/1 -> Bus Creator/2  "EcuBrk_tqEffBrkAxFrDes"
  Bus Creator/1 -> EcuBrk_Bus/1

== system Hybrid_vehicle/Vco (Vehicle Control)/EcuEdr (Electronic Control Unit for Edr) ==
  note: Vehicle Control Unit for Edr
  Edr_nEdr : Inport
  EcuGbxRe_tqEffEdrDes : Inport  Port=2
  Bus Creator : BusCreator  Inputs=1
  Gain : Gain  Gain=-1
  Ice_relLoadMax_CUR : Lookup_n-D  NumberOfTableDimensions=1  BreakpointsForDimension1=Edr_rpm_MaxMinTq_AXIS  Table=Edr_tqEffMax_CUR  ExtrapMethod=Clip  InternalRulePriority=Speed  RndMeth=Simplest  InputSameDT=on
  Max : MinMax  Function=max  Inputs=2
  Min : MinMax  Inputs=2
  Scope Edr : Scope  NumInputPorts=2
  EcuEdr_Bus : Outport  VectorParamsAs1DForOutWhenUnconnected=off
  wires:
  Bus Creator/1 -> EcuEdr_Bus/1
  Min/1 -> Max/1
  EcuGbxRe_tqEffEdrDes/1 -> Min/1  "EcuGbxRe_tqEffEdrDes"
  Max/1 -> Scope Edr/2, Bus Creator/1  "EcuEdr_tqEffEdrDes"
  Ice_relLoadMax_CUR/1 -> Min/2, Gain/1
  Gain/1 -> Max/2
  Edr_nEdr/1 -> Ice_relLoadMax_CUR/1, Scope Edr/1  "Edr_nEdr"

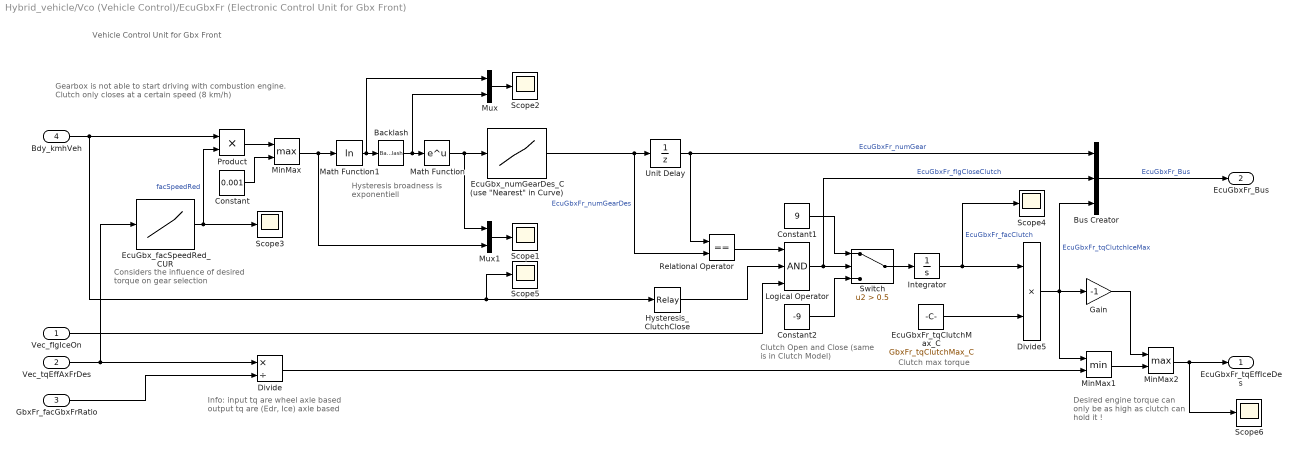
== system Hybrid_vehicle/Vco (Vehicle Control)/EcuGbxFr (Electronic Control Unit for Gbx Front) ==
  note: Gearbox is not able to start driving with combustion engine.
      | Clutch only closes at a certain speed (8 km/h)
  note: Vehicle Control Unit for Gbx Front
  note: Info:
      | input tq are wheel axle based
      | output tq are (Edr, Ice) axle based
  note: Considers the influence of
      | desired torque on gear selection
  note: Hysteresis broadness
      | is exponentiell
  note: Clutch Open and Close
      | (same is in Clutch Model)
  note: Desired engine torque can
      | only be as high as clutch
      | can hold it !
  note: Clutch max torque
  Vec_flgIceOn : Inport
  Vec_tqEffAxFrDes : Inport  Port=2
  GbxFr_facGbxFrRatio : Inport  Port=3
  Bdy_kmhVeh : Inport  Port=4
  Backlash : Backlash  BacklashWidth=0.5  InitialOutput=0.5
  Bus Creator : BusCreator  Inputs=3
  Constant : Constant  Value=0.001
  Constant1 : Constant  Value=9
  Constant2 : Constant  Value=-9
  Divide : Product  Inputs=*/
  Divide5 : Product  Inputs=**
  EcuGbxFr_tqClutchMax_C : Constant  Value=GbxFr_tqClutchMax_C
  EcuGbx_facSpeedRed_CUR : Lookup_n-D  NumberOfTableDimensions=1  BreakpointsForDimension1="[0  50  100 200 300 400 500]"  Table="[1.10  1.03  0.98  0.9  0.85  0.8  0.8 ]"  InternalRulePriority=Speed  RndMeth=Simplest  InputSameDT=on
  "EcuGbx_numGearDes_C (use \"Nearest\" in Curve) " : Lookup_n-D  NumberOfTableDimensions=1  BreakpointsForDimension1="[-0.1  14 25    35     55    80  90  ]"  Table="[1   1         2              3            4          5   5 ]"  InterpMethod=Nearest  InternalRulePriority=Speed  RndMeth=Simplest  InputSameDT=on
  Gain : Gain  Gain=-1
  Hysteresis_ClutchClose : Relay  OnSwitchValue=8  OffSwitchValue=7.5
  Integrator : Integrator  LimitOutput=on  UpperSaturationLimit=1  LowerSaturationLimit=0
  Logical Operator : Logic  Inputs=3  AllPortsSameDT=off  OutDataTypeStr=boolean
  Math Function : Math  SignedPower=on  SaturateOnIntegerOverflow=on
  Math Function1 : Math  Operator=log  SignedPower=on  SaturateOnIntegerOverflow=on
  MinMax : MinMax  Function=max  Inputs=2
  MinMax1 : MinMax  Inputs=2
  MinMax2 : MinMax  Function=max  Inputs=2
  Mux : Mux  Inputs=2
  Mux1 : Mux  Inputs=2
  Product : Product
  Relational Operator : RelationalOperator  Operator===  OutDataTypeStr=boolean  RndMeth=Simplest
  Scope{1..6} (6 alike) : Scope
  Switch : Switch  Criteria=u2 > Threshold  Threshold=0.5
  Unit Delay : UnitDelay  SampleTime=0.2  HasFrameUpgradeWarning=on
  EcuGbxFr_tqEffIceDes : Outport  VectorParamsAs1DForOutWhenUnconnected=off
  EcuGbxFr_Bus : Outport  Port=2  VectorParamsAs1DForOutWhenUnconnected=off
  wires:
  Bus Creator/1 -> EcuGbxFr_Bus/1  "EcuGbxFr_Bus"
  Vec_tqEffAxFrDes/1 -> Divide/1, EcuGbx_facSpeedRed_CUR/1
  Divide/1 -> MinMax1/2
  GbxFr_facGbxFrRatio/1 -> Divide/2
  "EcuGbx_numGearDes_C (use \"Nearest\" in Curve) "/1 -> Relational Operator/2, Unit Delay/1  "EcuGbxFr_numGearDes"
  Backlash/1 -> Mux/2, Math Function/1
  Bdy_kmhVeh/1 -> Hysteresis_ClutchClose/1, Scope5/1, Product/1
  Math Function1/1 -> Mux/1, Backlash/1
  EcuGbx_facSpeedRed_CUR/1 -> Scope3/1, Product/2  "facSpeedRed"
  MinMax/1 -> Math Function1/1, Mux1/2
  Math Function/1 -> Mux1/1, "EcuGbx_numGearDes_C (use \"Nearest\" in Curve) "/1
  Mux/1 -> Scope2/1
  Mux1/1 -> Scope1/1
  Product/1 -> MinMax/1
  Constant/1 -> MinMax/2
  Unit Delay/1 -> Bus Creator/1, Relational Operator/1  "EcuGbxFr_numGear"
  Constant1/1 -> Switch/1
  Switch/1 -> Integrator/1
  Logical Operator/1 -> Bus Creator/2, Switch/2  "EcuGbxFr_flgCloseClutch"
  Constant2/1 -> Switch/3
  Relational Operator/1 -> Logical Operator/1
  Hysteresis_ClutchClose/1 -> Logical Operator/2
  Integrator/1 -> Scope4/1, Divide5/1  "EcuGbxFr_facClutch"
  EcuGbxFr_tqClutchMax_C/1 -> Divide5/2
  Divide5/1 -> Gain/1, MinMax1/1, Bus Creator/3  "EcuGbxFr_tqClutchIceMax"
  MinMax2/1 -> EcuGbxFr_tqEffIceDes/1, Scope6/1
  MinMax1/1 -> MinMax2/2
  Gain/1 -> MinMax2/1
  Vec_flgIceOn/1 -> Logical Operator/3

== system Hybrid_vehicle/Vco (Vehicle Control)/EcuGbxRe (Electronic Control Unit for Gbx Rear) ==
  note: Vehicle Control Unit for Gbx Front
  note: Info:
      | input tq are wheel axle based
      | output tq are (Edr, Ice) axle based
  Vec_tqEffAxReDes : Inport
  GbxRe_facGbxReRatio : Inport  Port=2
  Bus Creator : BusCreator  Inputs=1
  Divide : Product  Inputs=*/
  EcuGbxRe_tqEffEdrDes : Outport  VectorParamsAs1DForOutWhenUnconnected=off
  EcuGbxRe_Bus : Outport  Port=2  VectorParamsAs1DForOutWhenUnconnected=off
  wires:
  Bus Creator/1 -> EcuGbxRe_Bus/1  "EcuGbxRe_Bus"
  Vec_tqEffAxReDes/1 -> Divide/1
  GbxRe_facGbxReRatio/1 -> Divide/2
  Divide/1 -> EcuGbxRe_tqEffEdrDes/1
  ? -> Bus Creator/1  "test"
